simulink model "Hexa_interface"  (R2023a)
settings: Solver=ode4  StartTime=0.0  StopTime=200  FixedStep=0.01  RelTol=1e-3
settings Model: Creator=danie  LastModifiedBy=danie

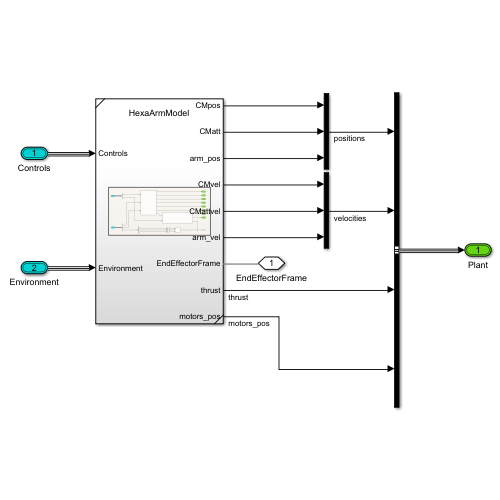
[thumbnail: Simulink's stored preview of the top-level diagram]
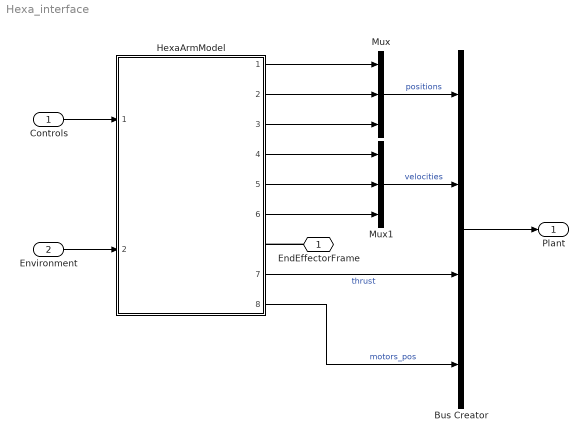
== system Hexa_interface ==
  Controls : Inport  OutDataTypeStr=Bus: ControlsBusDef
  Environment : Inport  Port=2  OutDataTypeStr=Bus: EnvironmentBusDef
  Bus Creator : BusCreator  Inputs=4
  HexaArmModel : Subsystem  ReferencedSubsystem=HexaArmModel
      settings: PortSchema="{\"entries\":[{\"content\":{\"sides\":[{\"content\":{\"connectorIds\":[\"In1\",\"In2\"]},\"type\":\"ConnectorPlacement.EquallySpacedRectSide\",\"uuid\":\"2dc8ce6a-8c2d-483c-b9eb-4519b8adf1d0\"},{\"content\":{\"connectorIds\":[\"Out1\",\"Out2\",\"Out3\",\"Out4\",\"Out5\",\"Out6\",\"LConn1\",\"Out7\",\"Out8\"],\"side\":\"RIGHT\"},\"type\":\"ConnectorPlacement.EquallySpacedRectSide\",\"uuid\":\"8919d7d9-a4a6-435e-91a0-6baaf43bb5dd\"},{\"content\":{\"side\":\"TOP\"},\"type\":\"ConnectorPlacement.EquallySpacedRectSide\",\"uuid\":\"fa3a5bef-28de-4da0-87cc-ec475f477ce4\"},{\"content\":{\"side\":\"BOTTOM\"},\"type\":\"ConnectorPlacement.EquallySpacedRectSide\",\"uuid\":\"150f6a32-8ea9-4dd2-b567-bcfc66bb4dd6\"}]},\"type\":\"ConnectorPlacement.EquallySpacedConnector\",\"uuid\":\"31c51f19-2717-4f79-8154-231ed584b48f\"}],\"packageUris\":[\"http://schema.mathworks.com/mf0/Connector/R2020b\"],\"version\":\"1.0\"}"
  Mux : Mux  Inputs=3
  Mux1 : Mux  Inputs=3
  EndEffectorFrame : PMIOPort  Side=Right
  Plant : Outport  OutDataTypeStr=Bus: PlantBusDef
  wires:
  HexaArmModel/8 -> Bus Creator/4  "motors_pos"
  HexaArmModel/5 -> Mux1/2
  Environment/1 -> HexaArmModel/2
  Mux1/1 -> Bus Creator/2  "velocities"
  HexaArmModel/7 -> Bus Creator/3  "thrust"
  Mux/1 -> Bus Creator/1  "positions"
  HexaArmModel/6 -> Mux1/3
  HexaArmModel/3 -> Mux/3
  HexaArmModel/2 -> Mux/2
  HexaArmModel/1 -> Mux/1
  Controls/1 -> HexaArmModel/1
  Bus Creator/1 -> Plant/1
  HexaArmModel/4 -> Mux1/1
  connections:
  EndEffectorFrame/RConn1 -- HexaArmModel/LConn1
